simulink model "Assignment3_2_MMC"  (R2024b)
settings: Solver=VariableStepAuto  StartTime=0.0  StopTime=0.35  MaxStep=1e-5  RelTol=1e-3
values from neighbouring files (symbols this model uses):
  C_sm = 5e-3    (= 0.005)    [assignment3.m]    (also in matlab.mat)
libraries: spsIGBTDiodeLib x48, spsSeriesRLCBranchLib x30, spsVoltageMeasurementLib x25, spsTriangleGeneratorLib x24, spsCurrentMeasurementLib x9, slpidlib x5, spsabctodq0Lib x3, spsdq0toabcLib x2, spsDCVoltageSourceLib x1, eePowerMeasurement x1, spsThreePhaseSeriesRLCBranchLib x1, spsThreePhaseVIMeasurementLib x1
(part 1 of 2)
settings Model: Creator=alexapf.stu  LastModifiedBy=alexapf.stu
settings SolverCC: ZeroCrossAlgorithm=Adaptive
settings DebuggingCC: IgnoredZcDiagnostic=none

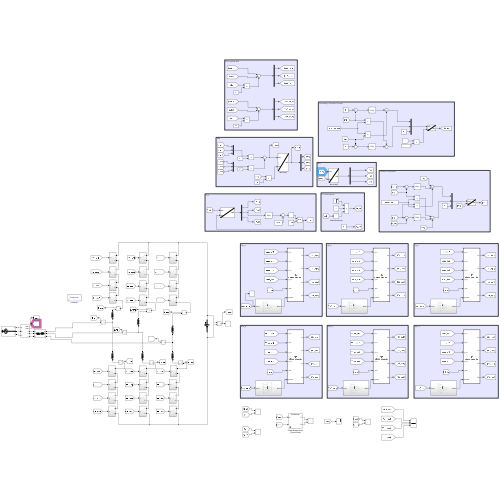
[thumbnail: Simulink's stored preview of the top-level diagram]
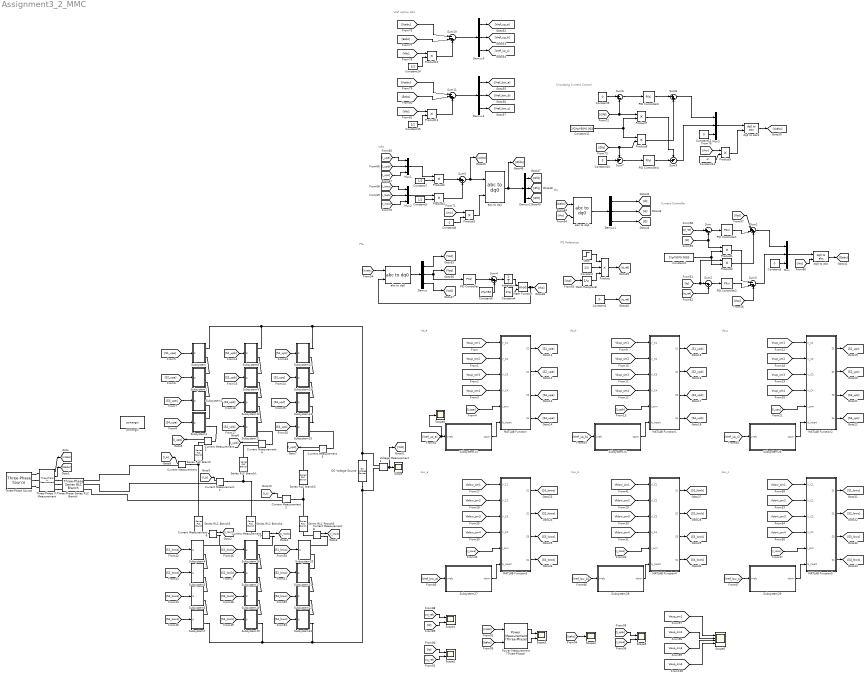
== system Assignment3_2_MMC ==
  note: Vref up/low abc
  note: Circulating Current Control
  note: izdq
  note: Idq
  note: Current Controller
  note: PQ Reference
  note: PLL
  note: Up_a
  note: Up_b
  note: Up_c
  note: low_c
  note: low_a
  note: low_b
  Constant : Constant  Value=2/3
  Constant{1,3,9..10,12} (5 alike) : Constant  Value=0
  Constant11 : Constant  Value=2*2*pi*50*0.003
  Constant13 : Constant  Value=-2
  Constant{5,7,14..15} (4 alike) : Constant  Value=1/2
  Constant2 : Constant  Value=2*pi*50*0.0083
  Constant4 : Constant  Value=2*pi
  Constant6 : Constant  Value=2*pi*50
  Constant8 : Constant  Value=-2
  Current Measurement{,1..8} (9 alike) : spsCurrentMeasurementLib/Current Measurement  PhasorSimulation=off  OutputType=Complex  PSBequivalent=0
  DC Voltage Source : spsDCVoltageSourceLib/DC Voltage Source  Amplitude=8e3  Measurements=None
  Demux{,1..4} (5 alike) : Demux  Outputs=3
  Integrator : Integrator
  MATLAB Function : MATLAB Function  TreatAsAtomicUnit=on
  MATLAB Function1 : MATLAB Function  TreatAsAtomicUnit=on
  MATLAB Function2 : MATLAB Function  TreatAsAtomicUnit=on
  MATLAB Function3 : MATLAB Function  TreatAsAtomicUnit=on
  MATLAB Function4 : MATLAB Function  TreatAsAtomicUnit=on
  MATLAB Function5 : MATLAB Function  TreatAsAtomicUnit=on
  Math Function : Math  Operator=mod
  Math Reciprocal : Math  Operator=reciprocal  SignedPower=on
  Mux{,1..3} (4 alike) : Mux  Inputs=3
  PID Controller : slpidlib/PID Controller  Controller=PI  Form=Parallel  TimeDomain=Continuous-time  UseExternalTs=off  SampleTime=-1  IntegratorMethod=Forward Euler  FilterMethod=Forward Euler  ControllerParametersSource=internal  P=0.0267  I=1.099  UseKiTs=off  D=0  UseExternalDerivativeSource=off  N=100  UseFilter=on  TunerSelectOption=Transfer Function Based (PID Tuner App)  InitialConditionSource=internal  InitialConditionForIntegrator=0  InitialConditionForFilter=0  DifferentiatorICPrevScaledInput=0  ExternalReset=none  TrackingMode=off  Kt=1  LimitOutput=off  SatLimitsSource=internal  UpperSaturationLimit=inf  LowerSaturationLimit=-inf  LinearizeAsGain=on  AntiWindupMode=none  Kb=1  LimitIntegrator=off  UpperIntegratorSaturationLimit=inf  LowerIntegratorSaturationLimit=-inf  POutMin=[]  POutMax=[]  IOutMin=[]  IOutMax=[]  DOutMin=[]  DOutMax=[]  NOutMin=[]  NOutMax=[]  SumOutMin=[]  SumOutMax=[]  SaturationOutMin=[]  SaturationOutMax=[]  PParamMin=[]  PParamMax=[]  IParamMin=[]  IParamMax=[]  DParamMin=[]  DParamMax=[]  NParamMin=[]  NParamMax=[]  KbParamMin=[]  KbParamMax=[]  KtParamMin=[]  KtParamMax=[]  KbOutMin=[]  KbOutMax=[]  KtOutMin=[]  KtOutMax=[]  IntegratorOutMin=[]  IntegratorOutMax=[]  FilterOutMin=[]  FilterOutMax=[]  SumI1OutMin=[]  SumI1OutMax=[]  SumI2OutMin=[]  SumI2OutMax=[]  SumI3OutMin=[]  SumI3OutMax=[]  SumI4OutMin=[]  SumI4OutMax=[]  SumDOutMin=[]  SumDOutMax=[]  DifferentiatorOutMin=[]  DifferentiatorOutMax=[]  FilterDiffOutCoefMin=[]  FilterDiffOutCoefMax=[]  ReciprocalOutMin=[]  ReciprocalOutMax=[]  SumDenOutMin=[]  SumDenOutMax=[]  SumNumOutMin=[]  SumNumOutMax=[]  DivideOutMin=[]  DivideOutMax=[]  UdiffTsProdOutMin=[]  UdiffTsProdOutMax=[]  NTsProdOutMin=[]  NTsProdOutMax=[]  UintegralTsProdOutMin=[]  UintegralTsProdOutMax=[]  UngainTsProdOutMin=[]  UngainTsProdOutMax=[]  ClampingZeroOutDataTypeStr=Inherit: Inherit via back propagation  ClampingZeroOutMin=[]  ClampingZeroOutMax=[]  FilterDenConstantOutDataTypeStr=Inherit: Inherit via back propagation  FilterDenConstantOutMin=[]  FilterDenConstantOutMax=[]  PCopyOutDataTypeStr=Inherit: Inherit via back propagation  PCopyOutMin=[]  PCopyOutMax=[]  NCopyOutDataTypeStr=Inherit: Inherit via back propagation  NCopyOutMin=[]  NCopyOutMax=[]  IntegratorContinuousStateAttributes=''  IntegratorStateMustResolveToSignalObject=off  IntegratorRTWStateStorageClass=Auto  FilterContinuousStateAttributes=''  FilterStateMustResolveToSignalObject=off  FilterRTWStateStorageClass=Auto  ParallelPVariant=InternalParameters  IdealPVariant=Disabled  IVariant=InternalParameters  DVariant=Disabled  IntegratorVariant=Continuous  SatVariant=Disabled  AWVariant=Passthrough  PCopyVariant=Disabled  TRVariant=Disabled  FdbkBlocksVariant=Forward  IdealPFdbkVariant=Disabled  SatFdbkVariant=Disabled  DerivativeFilterVariant=Disabled  NVariant=Disabled  NCopyVariant=Disabled_SignalSpec  FilterICVariant=Disabled  IntegratorICVariant=InternalICs  ExternalResetVariant=Disabled  TRSumVariant=Passthrough  SumFdbkVariant=Disabled  SumVariant=Sum_PI  TsampFilterVariant=InternalTs  TsampNgainVariant=Passthrough  TsampIntegralVariant=Disabled_SignalSpec  ExternalSaturationOutDataTypeStr=Inherit: Same as second input  DerivativeSourceVariant=Disabled  PreIntVariant=InternalPreInt
  PID Controller1 : slpidlib/PID Controller  Controller=PI  Form=Parallel  TimeDomain=Continuous-time  UseExternalTs=off  SampleTime=-1  IntegratorMethod=Forward Euler  FilterMethod=Forward Euler  ControllerParametersSource=internal  P=7.53  I=5.53  UseKiTs=off  D=0  UseExternalDerivativeSource=off  N=100  UseFilter=on  TunerSelectOption=Transfer Function Based (PID Tuner App)  InitialConditionSource=internal  InitialConditionForIntegrator=0  InitialConditionForFilter=0  DifferentiatorICPrevScaledInput=0  ExternalReset=none  TrackingMode=off  Kt=1  LimitOutput=off  SatLimitsSource=internal  UpperSaturationLimit=inf  LowerSaturationLimit=-inf  LinearizeAsGain=on  AntiWindupMode=none  Kb=1  LimitIntegrator=off  UpperIntegratorSaturationLimit=inf  LowerIntegratorSaturationLimit=-inf  POutMin=[]  POutMax=[]  IOutMin=[]  IOutMax=[]  DOutMin=[]  DOutMax=[]  NOutMin=[]  NOutMax=[]  SumOutMin=[]  SumOutMax=[]  SaturationOutMin=[]  SaturationOutMax=[]  PParamMin=[]  PParamMax=[]  IParamMin=[]  IParamMax=[]  DParamMin=[]  DParamMax=[]  NParamMin=[]  NParamMax=[]  KbParamMin=[]  KbParamMax=[]  KtParamMin=[]  KtParamMax=[]  KbOutMin=[]  KbOutMax=[]  KtOutMin=[]  KtOutMax=[]  IntegratorOutMin=[]  IntegratorOutMax=[]  FilterOutMin=[]  FilterOutMax=[]  SumI1OutMin=[]  SumI1OutMax=[]  SumI2OutMin=[]  SumI2OutMax=[]  SumI3OutMin=[]  SumI3OutMax=[]  SumI4OutMin=[]  SumI4OutMax=[]  SumDOutMin=[]  SumDOutMax=[]  DifferentiatorOutMin=[]  DifferentiatorOutMax=[]  FilterDiffOutCoefMin=[]  FilterDiffOutCoefMax=[]  ReciprocalOutMin=[]  ReciprocalOutMax=[]  SumDenOutMin=[]  SumDenOutMax=[]  SumNumOutMin=[]  SumNumOutMax=[]  DivideOutMin=[]  DivideOutMax=[]  UdiffTsProdOutMin=[]  UdiffTsProdOutMax=[]  NTsProdOutMin=[]  NTsProdOutMax=[]  UintegralTsProdOutMin=[]  UintegralTsProdOutMax=[]  UngainTsProdOutMin=[]  UngainTsProdOutMax=[]  ClampingZeroOutDataTypeStr=Inherit: Inherit via back propagation  ClampingZeroOutMin=[]  ClampingZeroOutMax=[]  FilterDenConstantOutDataTypeStr=Inherit: Inherit via back propagation  FilterDenConstantOutMin=[]  FilterDenConstantOutMax=[]  PCopyOutDataTypeStr=Inherit: Inherit via back propagation  PCopyOutMin=[]  PCopyOutMax=[]  NCopyOutDataTypeStr=Inherit: Inherit via back propagation  NCopyOutMin=[]  NCopyOutMax=[]  IntegratorContinuousStateAttributes=''  IntegratorStateMustResolveToSignalObject=off  IntegratorRTWStateStorageClass=Auto  FilterContinuousStateAttributes=''  FilterStateMustResolveToSignalObject=off  FilterRTWStateStorageClass=Auto  ParallelPVariant=InternalParameters  IdealPVariant=Disabled  IVariant=InternalParameters  DVariant=Disabled  IntegratorVariant=Continuous  SatVariant=Disabled  AWVariant=Passthrough  PCopyVariant=Disabled  TRVariant=Disabled  FdbkBlocksVariant=Forward  IdealPFdbkVariant=Disabled  SatFdbkVariant=Disabled  DerivativeFilterVariant=Disabled  NVariant=Disabled  NCopyVariant=Disabled_SignalSpec  FilterICVariant=Disabled  IntegratorICVariant=InternalICs  ExternalResetVariant=Disabled  TRSumVariant=Passthrough  SumFdbkVariant=Disabled  SumVariant=Sum_PI  TsampFilterVariant=InternalTs  TsampNgainVariant=Passthrough  TsampIntegralVariant=Disabled_SignalSpec  ExternalSaturationOutDataTypeStr=Inherit: Same as second input  DerivativeSourceVariant=Disabled  PreIntVariant=InternalPreInt
  PID Controller2 : slpidlib/PID Controller  Controller=PI  Form=Parallel  TimeDomain=Continuous-time  UseExternalTs=off  SampleTime=-1  IntegratorMethod=Forward Euler  FilterMethod=Forward Euler  ControllerParametersSource=internal  P=7.53  I=5.53  UseKiTs=off  D=0  UseExternalDerivativeSource=off  N=100  UseFilter=on  TunerSelectOption=Transfer Function Based (PID Tuner App)  InitialConditionSource=internal  InitialConditionForIntegrator=0  InitialConditionForFilter=0  DifferentiatorICPrevScaledInput=0  ExternalReset=none  TrackingMode=off  Kt=1  LimitOutput=off  SatLimitsSource=internal  UpperSaturationLimit=inf  LowerSaturationLimit=-inf  LinearizeAsGain=on  AntiWindupMode=none  Kb=1  LimitIntegrator=off  UpperIntegratorSaturationLimit=inf  LowerIntegratorSaturationLimit=-inf  POutMin=[]  POutMax=[]  IOutMin=[]  IOutMax=[]  DOutMin=[]  DOutMax=[]  NOutMin=[]  NOutMax=[]  SumOutMin=[]  SumOutMax=[]  SaturationOutMin=[]  SaturationOutMax=[]  PParamMin=[]  PParamMax=[]  IParamMin=[]  IParamMax=[]  DParamMin=[]  DParamMax=[]  NParamMin=[]  NParamMax=[]  KbParamMin=[]  KbParamMax=[]  KtParamMin=[]  KtParamMax=[]  KbOutMin=[]  KbOutMax=[]  KtOutMin=[]  KtOutMax=[]  IntegratorOutMin=[]  IntegratorOutMax=[]  FilterOutMin=[]  FilterOutMax=[]  SumI1OutMin=[]  SumI1OutMax=[]  SumI2OutMin=[]  SumI2OutMax=[]  SumI3OutMin=[]  SumI3OutMax=[]  SumI4OutMin=[]  SumI4OutMax=[]  SumDOutMin=[]  SumDOutMax=[]  DifferentiatorOutMin=[]  DifferentiatorOutMax=[]  FilterDiffOutCoefMin=[]  FilterDiffOutCoefMax=[]  ReciprocalOutMin=[]  ReciprocalOutMax=[]  SumDenOutMin=[]  SumDenOutMax=[]  SumNumOutMin=[]  SumNumOutMax=[]  DivideOutMin=[]  DivideOutMax=[]  UdiffTsProdOutMin=[]  UdiffTsProdOutMax=[]  NTsProdOutMin=[]  NTsProdOutMax=[]  UintegralTsProdOutMin=[]  UintegralTsProdOutMax=[]  UngainTsProdOutMin=[]  UngainTsProdOutMax=[]  ClampingZeroOutDataTypeStr=Inherit: Inherit via back propagation  ClampingZeroOutMin=[]  ClampingZeroOutMax=[]  FilterDenConstantOutDataTypeStr=Inherit: Inherit via back propagation  FilterDenConstantOutMin=[]  FilterDenConstantOutMax=[]  PCopyOutDataTypeStr=Inherit: Inherit via back propagation  PCopyOutMin=[]  PCopyOutMax=[]  NCopyOutDataTypeStr=Inherit: Inherit via back propagation  NCopyOutMin=[]  NCopyOutMax=[]  IntegratorContinuousStateAttributes=''  IntegratorStateMustResolveToSignalObject=off  IntegratorRTWStateStorageClass=Auto  FilterContinuousStateAttributes=''  FilterStateMustResolveToSignalObject=off  FilterRTWStateStorageClass=Auto  ParallelPVariant=InternalParameters  IdealPVariant=Disabled  IVariant=InternalParameters  DVariant=Disabled  IntegratorVariant=Continuous  SatVariant=Disabled  AWVariant=Passthrough  PCopyVariant=Disabled  TRVariant=Disabled  FdbkBlocksVariant=Forward  IdealPFdbkVariant=Disabled  SatFdbkVariant=Disabled  DerivativeFilterVariant=Disabled  NVariant=Disabled  NCopyVariant=Disabled_SignalSpec  FilterICVariant=Disabled  IntegratorICVariant=InternalICs  ExternalResetVariant=Disabled  TRSumVariant=Passthrough  SumFdbkVariant=Disabled  SumVariant=Sum_PI  TsampFilterVariant=InternalTs  TsampNgainVariant=Passthrough  TsampIntegralVariant=Disabled_SignalSpec  ExternalSaturationOutDataTypeStr=Inherit: Same as second input  DerivativeSourceVariant=Disabled  PreIntVariant=InternalPreInt
  PID Controller3 : slpidlib/PID Controller  Controller=PI  Form=Parallel  TimeDomain=Continuous-time  UseExternalTs=off  SampleTime=-1  IntegratorMethod=Forward Euler  FilterMethod=Forward Euler  ControllerParametersSource=internal  P=4  I=0  UseKiTs=off  D=0  UseExternalDerivativeSource=off  N=100  UseFilter=on  TunerSelectOption=Transfer Function Based (PID Tuner App)  InitialConditionSource=internal  InitialConditionForIntegrator=0  InitialConditionForFilter=0  DifferentiatorICPrevScaledInput=0  ExternalReset=none  TrackingMode=off  Kt=1  LimitOutput=off  SatLimitsSource=internal  UpperSaturationLimit=inf  LowerSaturationLimit=-inf  LinearizeAsGain=on  AntiWindupMode=none  Kb=1  LimitIntegrator=off  UpperIntegratorSaturationLimit=inf  LowerIntegratorSaturationLimit=-inf  POutMin=[]  POutMax=[]  IOutMin=[]  IOutMax=[]  DOutMin=[]  DOutMax=[]  NOutMin=[]  NOutMax=[]  SumOutMin=[]  SumOutMax=[]  SaturationOutMin=[]  SaturationOutMax=[]  PParamMin=[]  PParamMax=[]  IParamMin=[]  IParamMax=[]  DParamMin=[]  DParamMax=[]  NParamMin=[]  NParamMax=[]  KbParamMin=[]  KbParamMax=[]  KtParamMin=[]  KtParamMax=[]  KbOutMin=[]  KbOutMax=[]  KtOutMin=[]  KtOutMax=[]  IntegratorOutMin=[]  IntegratorOutMax=[]  FilterOutMin=[]  FilterOutMax=[]  SumI1OutMin=[]  SumI1OutMax=[]  SumI2OutMin=[]  SumI2OutMax=[]  SumI3OutMin=[]  SumI3OutMax=[]  SumI4OutMin=[]  SumI4OutMax=[]  SumDOutMin=[]  SumDOutMax=[]  DifferentiatorOutMin=[]  DifferentiatorOutMax=[]  FilterDiffOutCoefMin=[]  FilterDiffOutCoefMax=[]  ReciprocalOutMin=[]  ReciprocalOutMax=[]  SumDenOutMin=[]  SumDenOutMax=[]  SumNumOutMin=[]  SumNumOutMax=[]  DivideOutMin=[]  DivideOutMax=[]  UdiffTsProdOutMin=[]  UdiffTsProdOutMax=[]  NTsProdOutMin=[]  NTsProdOutMax=[]  UintegralTsProdOutMin=[]  UintegralTsProdOutMax=[]  UngainTsProdOutMin=[]  UngainTsProdOutMax=[]  ClampingZeroOutDataTypeStr=Inherit: Inherit via back propagation  ClampingZeroOutMin=[]  ClampingZeroOutMax=[]  FilterDenConstantOutDataTypeStr=Inherit: Inherit via back propagation  FilterDenConstantOutMin=[]  FilterDenConstantOutMax=[]  PCopyOutDataTypeStr=Inherit: Inherit via back propagation  PCopyOutMin=[]  PCopyOutMax=[]  NCopyOutDataTypeStr=Inherit: Inherit via back propagation  NCopyOutMin=[]  NCopyOutMax=[]  IntegratorContinuousStateAttributes=''  IntegratorStateMustResolveToSignalObject=off  IntegratorRTWStateStorageClass=Auto  FilterContinuousStateAttributes=''  FilterStateMustResolveToSignalObject=off  FilterRTWStateStorageClass=Auto  ParallelPVariant=InternalParameters  IdealPVariant=Disabled  IVariant=InternalParameters  DVariant=Disabled  IntegratorVariant=Continuous  SatVariant=Disabled  AWVariant=Passthrough  PCopyVariant=Disabled  TRVariant=Disabled  FdbkBlocksVariant=Forward  IdealPFdbkVariant=Disabled  SatFdbkVariant=Disabled  DerivativeFilterVariant=Disabled  NVariant=Disabled  NCopyVariant=Disabled_SignalSpec  FilterICVariant=Disabled  IntegratorICVariant=InternalICs  ExternalResetVariant=Disabled  TRSumVariant=Passthrough  SumFdbkVariant=Disabled  SumVariant=Sum_PI  TsampFilterVariant=InternalTs  TsampNgainVariant=Passthrough  TsampIntegralVariant=Disabled_SignalSpec  ExternalSaturationOutDataTypeStr=Inherit: Same as second input  DerivativeSourceVariant=Disabled  PreIntVariant=InternalPreInt
  PID Controller4 : slpidlib/PID Controller  Controller=PI  Form=Parallel  TimeDomain=Continuous-time  UseExternalTs=off  SampleTime=-1  IntegratorMethod=Forward Euler  FilterMethod=Forward Euler  ControllerParametersSource=internal  P=4  I=0  UseKiTs=off  D=0  UseExternalDerivativeSource=off  N=100  UseFilter=on  TunerSelectOption=Transfer Function Based (PID Tuner App)  InitialConditionSource=internal  InitialConditionForIntegrator=0  InitialConditionForFilter=0  DifferentiatorICPrevScaledInput=0  ExternalReset=none  TrackingMode=off  Kt=1  LimitOutput=off  SatLimitsSource=internal  UpperSaturationLimit=inf  LowerSaturationLimit=-inf  LinearizeAsGain=on  AntiWindupMode=none  Kb=1  LimitIntegrator=off  UpperIntegratorSaturationLimit=inf  LowerIntegratorSaturationLimit=-inf  POutMin=[]  POutMax=[]  IOutMin=[]  IOutMax=[]  DOutMin=[]  DOutMax=[]  NOutMin=[]  NOutMax=[]  SumOutMin=[]  SumOutMax=[]  SaturationOutMin=[]  SaturationOutMax=[]  PParamMin=[]  PParamMax=[]  IParamMin=[]  IParamMax=[]  DParamMin=[]  DParamMax=[]  NParamMin=[]  NParamMax=[]  KbParamMin=[]  KbParamMax=[]  KtParamMin=[]  KtParamMax=[]  KbOutMin=[]  KbOutMax=[]  KtOutMin=[]  KtOutMax=[]  IntegratorOutMin=[]  IntegratorOutMax=[]  FilterOutMin=[]  FilterOutMax=[]  SumI1OutMin=[]  SumI1OutMax=[]  SumI2OutMin=[]  SumI2OutMax=[]  SumI3OutMin=[]  SumI3OutMax=[]  SumI4OutMin=[]  SumI4OutMax=[]  SumDOutMin=[]  SumDOutMax=[]  DifferentiatorOutMin=[]  DifferentiatorOutMax=[]  FilterDiffOutCoefMin=[]  FilterDiffOutCoefMax=[]  ReciprocalOutMin=[]  ReciprocalOutMax=[]  SumDenOutMin=[]  SumDenOutMax=[]  SumNumOutMin=[]  SumNumOutMax=[]  DivideOutMin=[]  DivideOutMax=[]  UdiffTsProdOutMin=[]  UdiffTsProdOutMax=[]  NTsProdOutMin=[]  NTsProdOutMax=[]  UintegralTsProdOutMin=[]  UintegralTsProdOutMax=[]  UngainTsProdOutMin=[]  UngainTsProdOutMax=[]  ClampingZeroOutDataTypeStr=Inherit: Inherit via back propagation  ClampingZeroOutMin=[]  ClampingZeroOutMax=[]  FilterDenConstantOutDataTypeStr=Inherit: Inherit via back propagation  FilterDenConstantOutMin=[]  FilterDenConstantOutMax=[]  PCopyOutDataTypeStr=Inherit: Inherit via back propagation  PCopyOutMin=[]  PCopyOutMax=[]  NCopyOutDataTypeStr=Inherit: Inherit via back propagation  NCopyOutMin=[]  NCopyOutMax=[]  IntegratorContinuousStateAttributes=''  IntegratorStateMustResolveToSignalObject=off  IntegratorRTWStateStorageClass=Auto  FilterContinuousStateAttributes=''  FilterStateMustResolveToSignalObject=off  FilterRTWStateStorageClass=Auto  ParallelPVariant=InternalParameters  IdealPVariant=Disabled  IVariant=InternalParameters  DVariant=Disabled  IntegratorVariant=Continuous  SatVariant=Disabled  AWVariant=Passthrough  PCopyVariant=Disabled  TRVariant=Disabled  FdbkBlocksVariant=Forward  IdealPFdbkVariant=Disabled  SatFdbkVariant=Disabled  DerivativeFilterVariant=Disabled  NVariant=Disabled  NCopyVariant=Disabled_SignalSpec  FilterICVariant=Disabled  IntegratorICVariant=InternalICs  ExternalResetVariant=Disabled  TRSumVariant=Passthrough  SumFdbkVariant=Disabled  SumVariant=Sum_PI  TsampFilterVariant=InternalTs  TsampNgainVariant=Passthrough  TsampIntegralVariant=Disabled_SignalSpec  ExternalSaturationOutDataTypeStr=Inherit: Same as second input  DerivativeSourceVariant=Disabled  PreIntVariant=InternalPreInt
  Power Measurement (Three-Phase) : eePowerMeasurement/Power Measurement (Three-Phase)  LabelModeActiveChoice=Continuous  F=60  K=[1]  Seq=Positive  Ts=0
  Product : Product  Inputs=3
  Product{1..5,7..11} (10 alike) : Product
  Scope : Scope
  Scope{1..3,5} (4 alike) : Scope  NumInputPorts=2
  Scope4 : Scope
  Scope6 : Scope  NumInputPorts=4
  Scope8 : Scope
  Series RLC Branch{,1..5} (6 alike) : spsSeriesRLCBranchLib/Series RLC Branch  LConnTagsString=__new0  RConnTagsString=__new0  BranchType=L  Resistance=0  Inductance=3e-3  SetiL0=off  InitialCurrent=0  Capacitance=0  Setx0=off  InitialVoltage=0  Measurements=None
  Step : Step  Time=0.05  After=1e6  SampleTime=0.0001
  Subsystem : Subsystem
  Subsystem1 : Subsystem
  Subsystem10 : Subsystem
  Subsystem11 : Subsystem
  Subsystem12 : Subsystem
  Subsystem13 : Subsystem
  Subsystem14 : Subsystem
  Subsystem15 : Subsystem
  Subsystem16 : Subsystem
  Subsystem17 : Subsystem
  Subsystem18 : Subsystem
  Subsystem19 : Subsystem
  Subsystem2 : Subsystem
  Subsystem20 : Subsystem
  Subsystem21 : Subsystem
  Subsystem22 : Subsystem
  Subsystem23 : Subsystem
  Subsystem24 : Subsystem
  Subsystem25 : Subsystem
  Subsystem26 : Subsystem
  Subsystem27 : Subsystem
  Subsystem28 : Subsystem
  Subsystem29 : Subsystem
  Subsystem3 : Subsystem
  Subsystem4 : Subsystem
  Subsystem5 : Subsystem
  Subsystem6 : Subsystem
  Subsystem7 : Subsystem
  Subsystem8 : Subsystem
  Subsystem9 : Subsystem
  Sum : Sum  Inputs=|+-
  Sum1 : Sum  Inputs=|+-+
  Sum10 : Sum  Inputs=|--+
  Sum11 : Sum  Inputs=|-++
  Sum2 : Sum  Inputs=|-+
  Sum3 : Sum  Inputs=|--+
  Sum4 : Sum  Inputs=|++
  Sum5 : Sum  Inputs=|++
  Sum6 : Sum  Inputs=|+-
  Sum7 : Sum  Inputs=-+|
  Sum8 : Sum  Inputs=|++
  Sum9 : Sum  Inputs=-+|
  Three-Phase Series RLC Branch : spsThreePhaseSeriesRLCBranchLib/Three-Phase Series RLC Branch  LConnTagsString=A|B|C  RConnTagsString=A|B|C  BranchType=RL  Resistance=8.3e-3  Inductance=8.3e-3  Capacitance=1e-6  Measurements=Branch voltages and currents
  Three-Phase V-I Measurement : spsThreePhaseVIMeasurementLib/Three-Phase V-I Measurement  VoltageMeasurement=phase-to-ground  SetLabelV=off  LabelV=Vabc  Vpu=off  VpuLL=off  CurrentMeasurement=yes  SetLabelI=off  LabelI=Iabc  Ipu=off  Pbase=100e6  Vbase=500e3  OutputType=Complex  PhasorSimulation=off  PSBequivalent=0
  Three-Phase Source : spsThreePhaseSourceLib/Three-Phase Source  InternalConnection=Yg  VoltagePhases=off  Voltage=4160  PhaseAngle=0  Voltage_phases=[25e3 25e3 25e3]/sqrt(3)  PhaseAngles_phases=[0 -120 +120]  Frequency=50  NonIdealSource=off  SpecifyImpedance=off  Resistance=0.8929  Inductance=16.58e-3  ShortCircuitLevel=100e6  BaseVoltage=25e3  XRratio=7  BusType=swing  Pref=10e3  Qref=0  Prefabc=[10e3, 10e3, 10e3]  Qrefabc=[0, 0, 0]  Qmin=-inf  Qmax=inf
  Voltage Measurement3 : spsVoltageMeasurementLib/Voltage Measurement  PhasorSimulation=off  OutputType=Complex  PSBequivalent=0
  abc to dq0 : spsabctodq0Lib/abc to dq0  Alignment=90 degrees behind phase A axis
  abc to dq1 : spsabctodq0Lib/abc to dq0  Alignment=90 degrees behind phase A axis
  abc to dq2 : spsabctodq0Lib/abc to dq0  Alignment=90 degrees behind phase A axis
  dq0 to abc : spsdq0toabcLib/dq0 to abc  Alignment=90 degrees behind phase A axis
  dq0 to abc1 : spsdq0toabcLib/dq0 to abc  Alignment=90 degrees behind phase A axis
  powergui : spspowerguiLib/powergui  Priority=1  SimulationMode=Continuous  SampleTime=50e-6  frequency=60  Iterations=50  frequencyindice=50  Pbase=100e6  ErrMax=1e-4  UnitsV=kV  UnitsW=MW  buscounter=0  FunctionMessages=off  echomessages=off  EnableUseOfTLC=off  CurrentSourceSwitches=off  DisableSnubberDevices=off  DisableRonSwitches=off  DisableVfSwitches=off  DisplayEquations=off  AutomaticDiscreteSolvers=off  SolverType=Tustin/Backward Euler (TBE)  Interpol=off  ExternalGateDelay=off  methode=off  Ts=100  x0status=blocks  SPID=on  SwTol=0  HookPort=off  NonlinearTolerance=1e-4  nMaxIteration=100  ContinueOnMaxIteration=off  RestoreLinks=warning  ResistiveCurrentMeasurement=off  Frange=[0:2:500]  Ylog=off  Xlog=on  ShowGrid=off  save=off  variable=ZData  structure=0  ZoomFFT=off  StartTime=0.0  cycles=1  DisplayStyle=1  fundamental=60  FreqAxis=off  MaxFrequency=1000  frequencyindicesteady=1  RmsSteady=1  display=off
  wires:
  Three-Phase V-I Measurement/1 -> [Vsabc]
  Three-Phase V-I Measurement/2 -> [Isabc]
  Current Measurement6/1 -> [I_lowa]
  Current Measurement7/1 -> [I_lowb]
  Current Measurement8/1 -> [I_lowc]
  Current Measurement3/1 -> [I_upa]
  Current Measurement4/1 -> [I_upb]
  Current Measurement5/1 -> [I_upc]
  Current Measurement/1 -> [I_a]
  Current Measurement1/1 -> [I_b]
  Current Measurement2/1 -> [I_c]
  [S1_upa] -> Subsystem/1(g)
  [S2_upa] -> Subsystem1/1(g)
  [S3_upa] -> Subsystem2/1(g)
  [S4_upa] -> Subsystem3/1(g)
  [I_upa] -> MATLAB Function/5(i_arm)
  MATLAB Function/1(S1) -> [S1_upa]
  MATLAB Function/4(S4) -> [S4_upa]
  [Vaup_sm2] -> MATLAB Function/2(V_C2)
  [Vaup_sm4] -> MATLAB Function/4(V_C4)
  Subsystem24/1(Narm) -> MATLAB Function/6(N_insert)
  [Vaup_sm3] -> MATLAB Function/3(V_C3)
  [Vaup_sm1] -> MATLAB Function/1(V_C1)
  MATLAB Function/2(S2) -> [S2_upa]
  MATLAB Function/3(S3) -> [S3_upa]
  [Vref_up_a] -> Scope8/1, Subsystem24/1(Vref,j)
  [I_upb] -> MATLAB Function1/5(i_arm)
  [Vbup_sm2] -> MATLAB Function1/2(V_C2)
  [Vbup_sm4] -> MATLAB Function1/4(V_C4)
  Subsystem25/1(Narm) -> MATLAB Function1/6(N_insert)
  MATLAB Function1/1(S1) -> [S1_upb]
  [Vbup_sm3] -> MATLAB Function1/3(V_C3)
  MATLAB Function1/2(S2) -> [S2_upb]
  [Vbup_sm1] -> MATLAB Function1/1(V_C1)
  [Vref_up_b] -> Subsystem25/1(Vref,j)
  MATLAB Function1/4(S4) -> [S4_upb]
  MATLAB Function1/3(S3) -> [S3_upb]
  [S1_upb] -> Subsystem8/1(g)
  [S2_upb] -> Subsystem9/1(g)
  [S3_upb] -> Subsystem10/1(g)
  [S4_upb] -> Subsystem11/1(g)
  MATLAB Function2/4(S4) -> [S4_upc]
  [Vcup_sm2] -> MATLAB Function2/2(V_C2)
  MATLAB Function2/3(S3) -> [S3_upc]
  MATLAB Function2/1(S1) -> [S1_upc]
  [Vcup_sm1] -> MATLAB Function2/1(V_C1)
  Subsystem26/1(Narm) -> MATLAB Function2/6(N_insert)
  MATLAB Function2/2(S2) -> [S2_upc]
  [I_upc] -> MATLAB Function2/5(i_arm)
  [Vcup_sm3] -> MATLAB Function2/3(V_C3)
  [Vref_up_c] -> Subsystem26/1(Vref,j)
  [Vcup_sm4] -> MATLAB Function2/4(V_C4)
  [S1_upc] -> Subsystem12/1(g)
  [S2_upc] -> Subsystem13/1(g)
  [S3_upc] -> Subsystem14/1(g)
  [S4_upc] -> Subsystem15/1(g)
  [I_lowa] -> MATLAB Function3/5(i_arm)
  [Valow_sm2] -> MATLAB Function3/2(V_C2)
  Subsystem27/1(Narm) -> MATLAB Function3/6(N_insert)
  MATLAB Function3/1(S1) -> [S1_lowa]
  [Valow_sm3] -> MATLAB Function3/3(V_C3)
  MATLAB Function4/1(S1) -> [S1_lowb]
  Subsystem28/1(Narm) -> MATLAB Function4/6(N_insert)
  [Vclow_sm3] -> MATLAB Function5/3(V_C3)
  MATLAB Function4/3(S3) -> [S3_lowb]
  MATLAB Function5/2(S2) -> [S2_lowc]
  [Valow_sm4] -> MATLAB Function3/4(V_C4)
  [Vblow_sm4] -> MATLAB Function4/4(V_C4)
  [Vref_low_c] -> Subsystem29/1(Vref,j)
  MATLAB Function4/4(S4) -> [S4_lowb]
  [I_lowc] -> MATLAB Function5/5(i_arm)
  [Vblow_sm3] -> MATLAB Function4/3(V_C3)
  [Valow_sm1] -> MATLAB Function3/1(V_C1)
  MATLAB Function3/3(S3) -> [S3_lowa]
  [I_lowb] -> MATLAB Function4/5(i_arm)
  [Vblow_sm2] -> MATLAB Function4/2(V_C2)
  MATLAB Function3/2(S2) -> [S2_lowa]
  [Vref_low_b] -> Subsystem28/1(Vref,j)
  [Vblow_sm1] -> MATLAB Function4/1(V_C1)
  MATLAB Function4/2(S2) -> [S2_lowb]
  [Vclow_sm1] -> MATLAB Function5/1(V_C1)
  Subsystem29/1(Narm) -> MATLAB Function5/6(N_insert)
  MATLAB Function5/3(S3) -> [S3_lowc]
  [Vclow_sm2] -> MATLAB Function5/2(V_C2)
  MATLAB Function5/4(S4) -> [S4_lowc]
  MATLAB Function5/1(S1) -> [S1_lowc]
  [Vclow_sm4] -> MATLAB Function5/4(V_C4)
  [Vref_low_a] -> Subsystem27/1(Vref,j)
  MATLAB Function3/4(S4) -> [S4_lowa]
  [S2_lowa] -> Subsystem5/1(g)
  [S1_lowa] -> Subsystem4/1(g)
  [S4_lowa] -> Subsystem7/1(g)
  [S3_lowa] -> Subsystem6/1(g)
  [S2_lowb] -> Subsystem17/1(g)
  [S4_lowb] -> Subsystem19/1(g)
  [S1_lowb] -> Subsystem16/1(g)
  [S3_lowb] -> Subsystem18/1(g)
  [S1_lowc] -> Subsystem20/1(g)
  [S2_lowc] -> Subsystem21/1(g)
  [S3_lowc] -> Subsystem22/1(g)
  [S4_lowc] -> Subsystem23/1(g)
  Constant4/1 -> Math Function/2
  Constant6/1 -> Sum4/2
  [Vsabc] -> abc to dq0/1
  Demux/1 -> [Vsd]
  abc to dq0/1 -> Demux/1
  Demux/3 -> [Vs0]
  Sum4/1 -> Integrator/1
  PID Controller/1 -> Sum4/1
  Demux/2 -> [Vsq], PID Controller/1
  Integrator/1 -> Math Function/1
  Math Function/1 -> abc to dq0/2, [rho]
  Math Reciprocal/1 -> Product/3
  Step/1 -> Product/1
  Constant/1 -> Product/2
  Product/1 -> [Id_ref]
  [Vsd] -> Math Reciprocal/1
  Constant1/1 -> [Iq_ref]
  [rho] -> dq0 to abc/2
  [Vsd] -> Sum1/1
  [Iq_ref] -> Sum2/2
  [Id_ref] -> Sum/1
  Sum1/1 -> Mux/1
  Product2/1 -> Sum1/3
  Sum2/1 -> PID Controller2/1
  Constant3/1 -> Mux/3
  [Id] -> Product1/1, Sum/2
  Product1/1 -> Sum3/1
  Sum/1 -> PID Controller1/1
  Sum3/1 -> Mux/2
  PID Controller2/1 -> Sum3/2
  Mux/1 -> dq0 to abc/1
  dq0 to abc/1 -> [Eabc]
  [Vsq] -> Sum3/3
  PID Controller1/1 -> Sum1/2
  Constant2/1 -> Product1/2, Product2/2
  [Iq] -> Product2/1, Sum2/1
  [rho] -> abc to dq2/2
  Demux1/1 -> [Id]
  abc to dq2/1 -> Demux1/1
  Demux1/3 -> [I0]
  [Isabc] -> abc to dq2/1
  Demux1/2 -> [Iq]
  [I_upa] -> Mux1/1
  [I_lowc] -> Mux2/3
  [I_lowa] -> Mux2/1
  [I_upb] -> Mux1/2
  [I_lowb] -> Mux2/2
  Mux2/1 -> Product4/1
  Mux1/1 -> Product3/1
  Constant8/1 -> Product5/2
  Constant7/1 -> Product3/2
  Sum5/1 -> [izabc], abc to dq1/1
  Product3/1 -> Sum5/1
  [I_upc] -> Mux1/3
  [rho] -> Product5/1
  Product5/1 -> abc to dq1/2
  abc to dq1/1 -> Demux2/1, [i2fdq]
  Constant5/1 -> Product4/2
  Product4/1 -> Sum5/2
  Demux2/1 -> [i2fd]
  Demux2/2 -> [i2fq]
  Demux2/3 -> [i2f0]
  Product8/1 -> Sum8/2
  Sum7/1 -> PID Controller4/1
  Sum9/1 -> Mux3/2
  Constant13/1 -> Product9/2
  dq0 to abc1/1 -> [Vzabc]
  Constant12/1 -> Mux3/3
  PID Controller3/1 -> Sum8/1
  Mux3/1 -> dq0 to abc1/1
  Product9/1 -> dq0 to abc1/2
  Constant9/1 -> Sum6/1
  [rho] -> Product9/1
  Sum6/1 -> PID Controller3/1
  [i2fd] -> Product7/1, Sum6/2
  Sum8/1 -> Mux3/1
  [i2fq] -> Sum7/1, Product8/2
  Voltage Measurement3/1 -> [Vdc], Scope/1
  Demux3/1 -> [Vref_up_a]
  Demux3/2 -> [Vref_up_b]
  [Eabc] -> Sum10/2
  [Vdc] -> Product11/1
  [Vzabc] -> Sum11/1
  Product11/1 -> Sum11/3
  [Eabc] -> Sum11/2
  Constant15/1 -> Product11/2
  Demux4/3 -> [Vref_low_c]
  Demux4/1 -> [Vref_low_a]
  Demux4/2 -> [Vref_low_b]
  [Vzabc] -> Sum10/1
  Sum11/1 -> Demux4/1
  Demux3/3 -> [Vref_up_c]
  Product10/1 -> Sum10/3
  Constant14/1 -> Product10/2
  [Vdc] -> Product10/1
  Sum10/1 -> Demux3/1
  [Id_ref] -> Scope1/1
  [Id] -> Scope1/2
  [Iq] -> Scope2/1
  [Iq_ref] -> Scope2/2
  [Vsabc] -> Power Measurement (Three-Phase)/1
  Power Measurement (Three-Phase)/1 -> Scope3/1
  Power Measurement (Three-Phase)/2 -> Scope3/2
  [Isabc] -> Power Measurement (Three-Phase)/2
  [izabc] -> Scope4/1
  [I_upa] -> Scope5/1
  [I_lowa] -> Scope5/2
  [Vaup_sm1] -> Scope6/1
  [Vaup_sm3] -> Scope6/3
  [Vaup_sm2] -> Scope6/2
  [Vaup_sm4] -> Scope6/4
  Constant11/1 -> Product8/1, Product7/2
  PID Controller4/1 -> Sum9/2
  Product7/1 -> Sum9/1
  Constant10/1 -> Sum7/2
  connections:
  Subsystem1/RConn1 -- Subsystem/RConn2
  Subsystem2/RConn1 -- Subsystem1/RConn2
  Subsystem3/RConn1 -- Subsystem2/RConn2
  Series RLC Branch5/LConn1 -- Current Measurement2/LConn1 -- Series RLC Branch2/RConn1
  Current Measurement/RConn1 -- Three-Phase Series RLC Branch/RConn1
  Subsystem9/RConn1 -- Subsystem8/RConn2
  Subsystem10/RConn1 -- Subsystem9/RConn2
  Subsystem11/RConn1 -- Subsystem10/RConn2
  Subsystem13/RConn1 -- Subsystem12/RConn2
  Subsystem14/RConn1 -- Subsystem13/RConn2
  Subsystem15/RConn1 -- Subsystem14/RConn2
  Subsystem5/RConn1 -- Subsystem4/RConn2
  Subsystem6/RConn1 -- Subsystem5/RConn2
  Subsystem7/RConn1 -- Subsystem6/RConn2
  Subsystem19/RConn1 -- Subsystem18/RConn2
  Subsystem17/RConn1 -- Subsystem16/RConn2
  Subsystem18/RConn1 -- Subsystem17/RConn2
  Subsystem23/RConn1 -- Subsystem22/RConn2
  Subsystem21/RConn1 -- Subsystem20/RConn2
  Subsystem22/RConn1 -- Subsystem21/RConn2
  DC Voltage Source/RConn1 -- Subsystem12/RConn1 -- Subsystem8/RConn1 -- Subsystem/RConn1 -- Voltage Measurement3/LConn1
  DC Voltage Source/LConn1 -- Voltage Measurement3/LConn2 -- Subsystem23/RConn2 -- Subsystem19/RConn2 -- Subsystem7/RConn2
  Three-Phase V-I Measurement/RConn3 -- Three-Phase Series RLC Branch/LConn3
  Three-Phase Source/RConn2 -- Three-Phase V-I Measurement/LConn2
  Three-Phase V-I Measurement/RConn2 -- Three-Phase Series RLC Branch/LConn2
  Three-Phase Source/RConn1 -- Three-Phase V-I Measurement/LConn1
  Three-Phase V-I Measurement/RConn1 -- Three-Phase Series RLC Branch/LConn1
  Three-Phase Source/RConn3 -- Three-Phase V-I Measurement/LConn3
  Series RLC Branch1/RConn1 -- Current Measurement1/LConn1 -- Series RLC Branch4/LConn1
  Series RLC Branch3/LConn1 -- Current Measurement/LConn1 -- Series RLC Branch/RConn1
  Current Measurement1/RConn1 -- Three-Phase Series RLC Branch/RConn2
  Current Measurement2/RConn1 -- Three-Phase Series RLC Branch/RConn3
  Subsystem3/RConn2 -- Current Measurement3/LConn1
  Current Measurement3/RConn1 -- Series RLC Branch/LConn1
  Current Measurement4/LConn1 -- Subsystem11/RConn2
  Current Measurement4/RConn1 -- Series RLC Branch1/LConn1
  Current Measurement5/LConn1 -- Subsystem15/RConn2
  Current Measurement5/RConn1 -- Series RLC Branch2/LConn1
  Current Measurement6/LConn1 -- Series RLC Branch3/RConn1
  Current Measurement6/RConn1 -- Subsystem4/RConn1
  Current Measurement7/LConn1 -- Series RLC Branch4/RConn1
  Current Measurement7/RConn1 -- Subsystem16/RConn1
  Series RLC Branch5/RConn1 -- Current Measurement8/LConn1
  Current Measurement8/RConn1 -- Subsystem20/RConn1

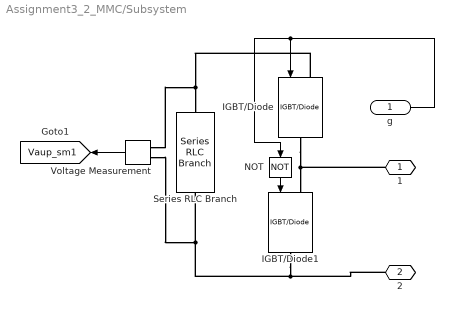
== system Assignment3_2_MMC/Subsystem ==
  g : Inport
  IGBT/Diode : spsIGBTDiodeLib/IGBT//Diode  Ron=1e-3  Rs=1e5  Cs=inf  Measurements=off
  IGBT/Diode1 : spsIGBTDiodeLib/IGBT//Diode  Ron=1e-3  Rs=1e5  Cs=inf  Measurements=off
  NOT : Logic  Operator=NOT  IconShape=distinctive  AllPortsSameDT=off  OutDataTypeStr=boolean
  Series RLC Branch : spsSeriesRLCBranchLib/Series RLC Branch  LConnTagsString=__new0  RConnTagsString=__new0  BranchType=C  Resistance=1  Inductance=1e-3  SetiL0=off  InitialCurrent=0  Capacitance=C_sm  Setx0=on  InitialVoltage=V_sm  Measurements=None
  Voltage Measurement : spsVoltageMeasurementLib/Voltage Measurement  PhasorSimulation=off  OutputType=Complex  PSBequivalent=0
  1 : PMIOPort  Side=Right
  2 : PMIOPort  Port=2  Side=Right
  tag scope: Vaup_sm1=global
  wires:
  NOT/1 -> IGBT/Diode1/1
  g/1 -> IGBT/Diode/1, NOT/1
  Voltage Measurement/1 -> [Vaup_sm1]
  connections:
  IGBT/Diode/RConn1 -- IGBT/Diode1/LConn1 -- 1/RConn1
  IGBT/Diode/LConn1 -- Voltage Measurement/LConn1 -- Series RLC Branch/LConn1
  IGBT/Diode1/RConn1 -- 2/RConn1 -- Voltage Measurement/LConn2 -- Series RLC Branch/RConn1

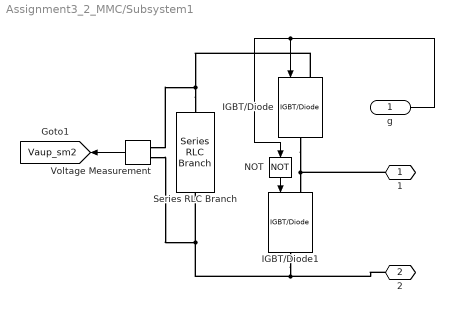
== system Assignment3_2_MMC/Subsystem1 ==
  g : Inport
  IGBT/Diode : spsIGBTDiodeLib/IGBT//Diode  Ron=1e-3  Rs=1e5  Cs=inf  Measurements=off
  IGBT/Diode1 : spsIGBTDiodeLib/IGBT//Diode  Ron=1e-3  Rs=1e5  Cs=inf  Measurements=off
  NOT : Logic  Operator=NOT  IconShape=distinctive  AllPortsSameDT=off  OutDataTypeStr=boolean
  Series RLC Branch : spsSeriesRLCBranchLib/Series RLC Branch  LConnTagsString=__new0  RConnTagsString=__new0  BranchType=C  Resistance=1  Inductance=1e-3  SetiL0=off  InitialCurrent=0  Capacitance=C_sm  Setx0=on  InitialVoltage=V_sm  Measurements=None
  Voltage Measurement : spsVoltageMeasurementLib/Voltage Measurement  PhasorSimulation=off  OutputType=Complex  PSBequivalent=0
  1 : PMIOPort  Side=Right
  2 : PMIOPort  Port=2  Side=Right
  tag scope: Vaup_sm2=global
  wires:
  NOT/1 -> IGBT/Diode1/1
  g/1 -> IGBT/Diode/1, NOT/1
  Voltage Measurement/1 -> [Vaup_sm2]
  connections:
  IGBT/Diode/RConn1 -- 1/RConn1 -- IGBT/Diode1/LConn1
  Series RLC Branch/LConn1 -- IGBT/Diode/LConn1 -- Voltage Measurement/LConn1
  Series RLC Branch/RConn1 -- 2/RConn1 -- IGBT/Diode1/RConn1 -- Voltage Measurement/LConn2

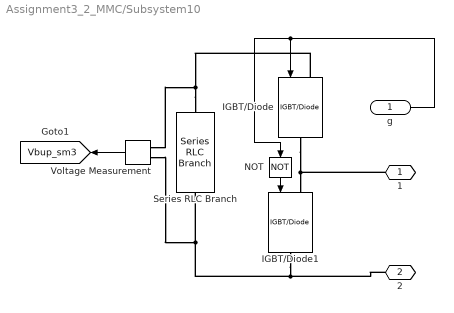
== system Assignment3_2_MMC/Subsystem10 ==
  g : Inport
  IGBT/Diode : spsIGBTDiodeLib/IGBT//Diode  Ron=1e-3  Rs=1e5  Cs=inf  Measurements=off
  IGBT/Diode1 : spsIGBTDiodeLib/IGBT//Diode  Ron=1e-3  Rs=1e5  Cs=inf  Measurements=off
  NOT : Logic  Operator=NOT  IconShape=distinctive  AllPortsSameDT=off  OutDataTypeStr=boolean
  Series RLC Branch : spsSeriesRLCBranchLib/Series RLC Branch  LConnTagsString=__new0  RConnTagsString=__new0  BranchType=C  Resistance=1  Inductance=1e-3  SetiL0=off  InitialCurrent=0  Capacitance=C_sm  Setx0=on  InitialVoltage=V_sm  Measurements=None
  Voltage Measurement : spsVoltageMeasurementLib/Voltage Measurement  PhasorSimulation=off  OutputType=Complex  PSBequivalent=0
  1 : PMIOPort  Side=Right
  2 : PMIOPort  Port=2  Side=Right
  tag scope: Vbup_sm3=global
  wires:
  NOT/1 -> IGBT/Diode1/1
  g/1 -> IGBT/Diode/1, NOT/1
  Voltage Measurement/1 -> [Vbup_sm3]
  connections:
  IGBT/Diode/RConn1 -- 1/RConn1 -- IGBT/Diode1/LConn1
  Series RLC Branch/LConn1 -- IGBT/Diode/LConn1 -- Voltage Measurement/LConn1
  Series RLC Branch/RConn1 -- 2/RConn1 -- IGBT/Diode1/RConn1 -- Voltage Measurement/LConn2

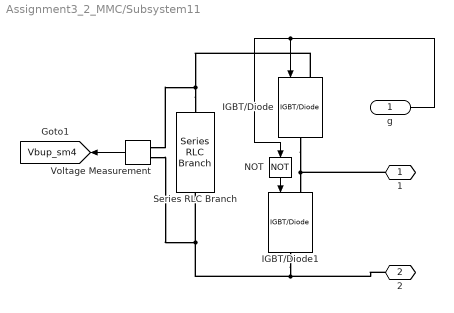
== system Assignment3_2_MMC/Subsystem11 ==
  g : Inport
  IGBT/Diode : spsIGBTDiodeLib/IGBT//Diode  Ron=1e-3  Rs=1e5  Cs=inf  Measurements=off
  IGBT/Diode1 : spsIGBTDiodeLib/IGBT//Diode  Ron=1e-3  Rs=1e5  Cs=inf  Measurements=off
  NOT : Logic  Operator=NOT  IconShape=distinctive  AllPortsSameDT=off  OutDataTypeStr=boolean
  Series RLC Branch : spsSeriesRLCBranchLib/Series RLC Branch  LConnTagsString=__new0  RConnTagsString=__new0  BranchType=C  Resistance=1  Inductance=1e-3  SetiL0=off  InitialCurrent=0  Capacitance=C_sm  Setx0=on  InitialVoltage=V_sm  Measurements=None
  Voltage Measurement : spsVoltageMeasurementLib/Voltage Measurement  PhasorSimulation=off  OutputType=Complex  PSBequivalent=0
  1 : PMIOPort  Side=Right
  2 : PMIOPort  Port=2  Side=Right
  tag scope: Vbup_sm4=global
  wires:
  NOT/1 -> IGBT/Diode1/1
  g/1 -> IGBT/Diode/1, NOT/1
  Voltage Measurement/1 -> [Vbup_sm4]
  connections:
  IGBT/Diode/RConn1 -- 1/RConn1 -- IGBT/Diode1/LConn1
  Series RLC Branch/LConn1 -- IGBT/Diode/LConn1 -- Voltage Measurement/LConn1
  Series RLC Branch/RConn1 -- 2/RConn1 -- IGBT/Diode1/RConn1 -- Voltage Measurement/LConn2

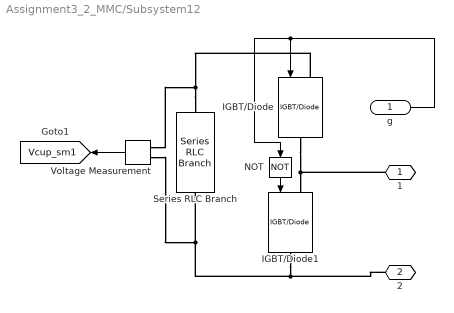
== system Assignment3_2_MMC/Subsystem12 ==
  g : Inport
  IGBT/Diode : spsIGBTDiodeLib/IGBT//Diode  Ron=1e-3  Rs=1e5  Cs=inf  Measurements=off
  IGBT/Diode1 : spsIGBTDiodeLib/IGBT//Diode  Ron=1e-3  Rs=1e5  Cs=inf  Measurements=off
  NOT : Logic  Operator=NOT  IconShape=distinctive  AllPortsSameDT=off  OutDataTypeStr=boolean
  Series RLC Branch : spsSeriesRLCBranchLib/Series RLC Branch  LConnTagsString=__new0  RConnTagsString=__new0  BranchType=C  Resistance=1  Inductance=1e-3  SetiL0=off  InitialCurrent=0  Capacitance=C_sm  Setx0=on  InitialVoltage=V_sm  Measurements=None
  Voltage Measurement : spsVoltageMeasurementLib/Voltage Measurement  PhasorSimulation=off  OutputType=Complex  PSBequivalent=0
  1 : PMIOPort  Side=Right
  2 : PMIOPort  Port=2  Side=Right
  tag scope: Vcup_sm1=global
  wires:
  NOT/1 -> IGBT/Diode1/1
  g/1 -> IGBT/Diode/1, NOT/1
  Voltage Measurement/1 -> [Vcup_sm1]
  connections:
  IGBT/Diode/RConn1 -- 1/RConn1 -- IGBT/Diode1/LConn1
  Series RLC Branch/LConn1 -- IGBT/Diode/LConn1 -- Voltage Measurement/LConn1
  Series RLC Branch/RConn1 -- 2/RConn1 -- IGBT/Diode1/RConn1 -- Voltage Measurement/LConn2

== system Assignment3_2_MMC/Subsystem13 ==
  g : Inport
  IGBT/Diode : spsIGBTDiodeLib/IGBT//Diode  Ron=1e-3  Rs=1e5  Cs=inf  Measurements=off
  IGBT/Diode1 : spsIGBTDiodeLib/IGBT//Diode  Ron=1e-3  Rs=1e5  Cs=inf  Measurements=off
  NOT : Logic  Operator=NOT  IconShape=distinctive  AllPortsSameDT=off  OutDataTypeStr=boolean
  Series RLC Branch : spsSeriesRLCBranchLib/Series RLC Branch  LConnTagsString=__new0  RConnTagsString=__new0  BranchType=C  Resistance=1  Inductance=1e-3  SetiL0=off  InitialCurrent=0  Capacitance=C_sm  Setx0=on  InitialVoltage=V_sm  Measurements=None
  Voltage Measurement : spsVoltageMeasurementLib/Voltage Measurement  PhasorSimulation=off  OutputType=Complex  PSBequivalent=0
  1 : PMIOPort  Side=Right
  2 : PMIOPort  Port=2  Side=Right
  tag scope: Vcup_sm2=global
  wires:
  NOT/1 -> IGBT/Diode1/1
  g/1 -> IGBT/Diode/1, NOT/1
  Voltage Measurement/1 -> [Vcup_sm2]
  connections:
  IGBT/Diode/RConn1 -- 1/RConn1 -- IGBT/Diode1/LConn1
  Series RLC Branch/LConn1 -- IGBT/Diode/LConn1 -- Voltage Measurement/LConn1
  Series RLC Branch/RConn1 -- 2/RConn1 -- IGBT/Diode1/RConn1 -- Voltage Measurement/LConn2

== system Assignment3_2_MMC/Subsystem14 ==
  g : Inport
  IGBT/Diode : spsIGBTDiodeLib/IGBT//Diode  Ron=1e-3  Rs=1e5  Cs=inf  Measurements=off
  IGBT/Diode1 : spsIGBTDiodeLib/IGBT//Diode  Ron=1e-3  Rs=1e5  Cs=inf  Measurements=off
  NOT : Logic  Operator=NOT  IconShape=distinctive  AllPortsSameDT=off  OutDataTypeStr=boolean
  Series RLC Branch : spsSeriesRLCBranchLib/Series RLC Branch  LConnTagsString=__new0  RConnTagsString=__new0  BranchType=C  Resistance=1  Inductance=1e-3  SetiL0=off  InitialCurrent=0  Capacitance=C_sm  Setx0=on  InitialVoltage=V_sm  Measurements=None
  Voltage Measurement : spsVoltageMeasurementLib/Voltage Measurement  PhasorSimulation=off  OutputType=Complex  PSBequivalent=0
  1 : PMIOPort  Side=Right
  2 : PMIOPort  Port=2  Side=Right
  tag scope: Vcup_sm3=global
  wires:
  NOT/1 -> IGBT/Diode1/1
  g/1 -> IGBT/Diode/1, NOT/1
  Voltage Measurement/1 -> [Vcup_sm3]
  connections:
  IGBT/Diode/RConn1 -- 1/RConn1 -- IGBT/Diode1/LConn1
  Series RLC Branch/LConn1 -- IGBT/Diode/LConn1 -- Voltage Measurement/LConn1
  Series RLC Branch/RConn1 -- 2/RConn1 -- IGBT/Diode1/RConn1 -- Voltage Measurement/LConn2

== system Assignment3_2_MMC/Subsystem15 ==
  g : Inport
  IGBT/Diode : spsIGBTDiodeLib/IGBT//Diode  Ron=1e-3  Rs=1e5  Cs=inf  Measurements=off
  IGBT/Diode1 : spsIGBTDiodeLib/IGBT//Diode  Ron=1e-3  Rs=1e5  Cs=inf  Measurements=off
  NOT : Logic  Operator=NOT  IconShape=distinctive  AllPortsSameDT=off  OutDataTypeStr=boolean
  Series RLC Branch : spsSeriesRLCBranchLib/Series RLC Branch  LConnTagsString=__new0  RConnTagsString=__new0  BranchType=C  Resistance=1  Inductance=1e-3  SetiL0=off  InitialCurrent=0  Capacitance=C_sm  Setx0=on  InitialVoltage=V_sm  Measurements=None
  Voltage Measurement : spsVoltageMeasurementLib/Voltage Measurement  PhasorSimulation=off  OutputType=Complex  PSBequivalent=0
  1 : PMIOPort  Side=Right
  2 : PMIOPort  Port=2  Side=Right
  tag scope: Vcup_sm4=global
  wires:
  NOT/1 -> IGBT/Diode1/1
  g/1 -> IGBT/Diode/1, NOT/1
  Voltage Measurement/1 -> [Vcup_sm4]
  connections:
  IGBT/Diode/RConn1 -- 1/RConn1 -- IGBT/Diode1/LConn1
  Series RLC Branch/LConn1 -- IGBT/Diode/LConn1 -- Voltage Measurement/LConn1
  Series RLC Branch/RConn1 -- 2/RConn1 -- IGBT/Diode1/RConn1 -- Voltage Measurement/LConn2

== system Assignment3_2_MMC/Subsystem16 ==
  g : Inport
  IGBT/Diode : spsIGBTDiodeLib/IGBT//Diode  Ron=1e-3  Rs=1e5  Cs=inf  Measurements=off
  IGBT/Diode1 : spsIGBTDiodeLib/IGBT//Diode  Ron=1e-3  Rs=1e5  Cs=inf  Measurements=off
  NOT : Logic  Operator=NOT  IconShape=distinctive  AllPortsSameDT=off  OutDataTypeStr=boolean
  Series RLC Branch : spsSeriesRLCBranchLib/Series RLC Branch  LConnTagsString=__new0  RConnTagsString=__new0  BranchType=C  Resistance=1  Inductance=1e-3  SetiL0=off  InitialCurrent=0  Capacitance=C_sm  Setx0=on  InitialVoltage=V_sm  Measurements=None
  Voltage Measurement : spsVoltageMeasurementLib/Voltage Measurement  PhasorSimulation=off  OutputType=Complex  PSBequivalent=0
  1 : PMIOPort  Side=Right
  2 : PMIOPort  Port=2  Side=Right
  tag scope: Vblow_sm1=global
  wires:
  NOT/1 -> IGBT/Diode1/1
  g/1 -> IGBT/Diode/1, NOT/1
  Voltage Measurement/1 -> [Vblow_sm1]
  connections:
  IGBT/Diode/RConn1 -- 1/RConn1 -- IGBT/Diode1/LConn1
  Series RLC Branch/LConn1 -- IGBT/Diode/LConn1 -- Voltage Measurement/LConn1
  Series RLC Branch/RConn1 -- 2/RConn1 -- IGBT/Diode1/RConn1 -- Voltage Measurement/LConn2

== system Assignment3_2_MMC/Subsystem17 ==
  g : Inport
  IGBT/Diode : spsIGBTDiodeLib/IGBT//Diode  Ron=1e-3  Rs=1e5  Cs=inf  Measurements=off
  IGBT/Diode1 : spsIGBTDiodeLib/IGBT//Diode  Ron=1e-3  Rs=1e5  Cs=inf  Measurements=off
  NOT : Logic  Operator=NOT  IconShape=distinctive  AllPortsSameDT=off  OutDataTypeStr=boolean
  Series RLC Branch : spsSeriesRLCBranchLib/Series RLC Branch  LConnTagsString=__new0  RConnTagsString=__new0  BranchType=C  Resistance=1  Inductance=1e-3  SetiL0=off  InitialCurrent=0  Capacitance=C_sm  Setx0=on  InitialVoltage=V_sm  Measurements=None
  Voltage Measurement : spsVoltageMeasurementLib/Voltage Measurement  PhasorSimulation=off  OutputType=Complex  PSBequivalent=0
  1 : PMIOPort  Side=Right
  2 : PMIOPort  Port=2  Side=Right
  tag scope: Vblow_sm2=global
  wires:
  NOT/1 -> IGBT/Diode1/1
  g/1 -> IGBT/Diode/1, NOT/1
  Voltage Measurement/1 -> [Vblow_sm2]
  connections:
  IGBT/Diode/RConn1 -- 1/RConn1 -- IGBT/Diode1/LConn1
  Series RLC Branch/LConn1 -- IGBT/Diode/LConn1 -- Voltage Measurement/LConn1
  Series RLC Branch/RConn1 -- 2/RConn1 -- IGBT/Diode1/RConn1 -- Voltage Measurement/LConn2

== system Assignment3_2_MMC/Subsystem18 ==
  g : Inport
  IGBT/Diode : spsIGBTDiodeLib/IGBT//Diode  Ron=1e-3  Rs=1e5  Cs=inf  Measurements=off
  IGBT/Diode1 : spsIGBTDiodeLib/IGBT//Diode  Ron=1e-3  Rs=1e5  Cs=inf  Measurements=off
  NOT : Logic  Operator=NOT  IconShape=distinctive  AllPortsSameDT=off  OutDataTypeStr=boolean
  Series RLC Branch : spsSeriesRLCBranchLib/Series RLC Branch  LConnTagsString=__new0  RConnTagsString=__new0  BranchType=C  Resistance=1  Inductance=1e-3  SetiL0=off  InitialCurrent=0  Capacitance=C_sm  Setx0=on  InitialVoltage=V_sm  Measurements=None
  Voltage Measurement : spsVoltageMeasurementLib/Voltage Measurement  PhasorSimulation=off  OutputType=Complex  PSBequivalent=0
  1 : PMIOPort  Side=Right
  2 : PMIOPort  Port=2  Side=Right
  tag scope: Vblow_sm3=global
  wires:
  NOT/1 -> IGBT/Diode1/1
  g/1 -> IGBT/Diode/1, NOT/1
  Voltage Measurement/1 -> [Vblow_sm3]
  connections:
  IGBT/Diode/RConn1 -- 1/RConn1 -- IGBT/Diode1/LConn1
  Series RLC Branch/LConn1 -- IGBT/Diode/LConn1 -- Voltage Measurement/LConn1
  Series RLC Branch/RConn1 -- 2/RConn1 -- IGBT/Diode1/RConn1 -- Voltage Measurement/LConn2

== system Assignment3_2_MMC/Subsystem19 ==
  g : Inport
  IGBT/Diode : spsIGBTDiodeLib/IGBT//Diode  Ron=1e-3  Rs=1e5  Cs=inf  Measurements=off
  IGBT/Diode1 : spsIGBTDiodeLib/IGBT//Diode  Ron=1e-3  Rs=1e5  Cs=inf  Measurements=off
  NOT : Logic  Operator=NOT  IconShape=distinctive  AllPortsSameDT=off  OutDataTypeStr=boolean
  Series RLC Branch : spsSeriesRLCBranchLib/Series RLC Branch  LConnTagsString=__new0  RConnTagsString=__new0  BranchType=C  Resistance=1  Inductance=1e-3  SetiL0=off  InitialCurrent=0  Capacitance=C_sm  Setx0=on  InitialVoltage=V_sm  Measurements=None
  Voltage Measurement : spsVoltageMeasurementLib/Voltage Measurement  PhasorSimulation=off  OutputType=Complex  PSBequivalent=0
  1 : PMIOPort  Side=Right
  2 : PMIOPort  Port=2  Side=Right
  tag scope: Vblow_sm4=global
  wires:
  NOT/1 -> IGBT/Diode1/1
  g/1 -> IGBT/Diode/1, NOT/1
  Voltage Measurement/1 -> [Vblow_sm4]
  connections:
  IGBT/Diode/RConn1 -- 1/RConn1 -- IGBT/Diode1/LConn1
  Series RLC Branch/LConn1 -- IGBT/Diode/LConn1 -- Voltage Measurement/LConn1
  Series RLC Branch/RConn1 -- 2/RConn1 -- IGBT/Diode1/RConn1 -- Voltage Measurement/LConn2

== system Assignment3_2_MMC/Subsystem2 ==
  g : Inport
  IGBT/Diode : spsIGBTDiodeLib/IGBT//Diode  Ron=1e-3  Rs=1e5  Cs=inf  Measurements=off
  IGBT/Diode1 : spsIGBTDiodeLib/IGBT//Diode  Ron=1e-3  Rs=1e5  Cs=inf  Measurements=off
  NOT : Logic  Operator=NOT  IconShape=distinctive  AllPortsSameDT=off  OutDataTypeStr=boolean
  Series RLC Branch : spsSeriesRLCBranchLib/Series RLC Branch  LConnTagsString=__new0  RConnTagsString=__new0  BranchType=C  Resistance=1  Inductance=1e-3  SetiL0=off  InitialCurrent=0  Capacitance=C_sm  Setx0=on  InitialVoltage=V_sm  Measurements=None
  Voltage Measurement : spsVoltageMeasurementLib/Voltage Measurement  PhasorSimulation=off  OutputType=Complex  PSBequivalent=0
  1 : PMIOPort  Side=Right
  2 : PMIOPort  Port=2  Side=Right
  tag scope: Vaup_sm3=global
  wires:
  NOT/1 -> IGBT/Diode1/1
  g/1 -> IGBT/Diode/1, NOT/1
  Voltage Measurement/1 -> [Vaup_sm3]
  connections:
  IGBT/Diode/RConn1 -- 1/RConn1 -- IGBT/Diode1/LConn1
  Series RLC Branch/LConn1 -- IGBT/Diode/LConn1 -- Voltage Measurement/LConn1
  Series RLC Branch/RConn1 -- 2/RConn1 -- IGBT/Diode1/RConn1 -- Voltage Measurement/LConn2

== system Assignment3_2_MMC/Subsystem20 ==
  g : Inport
  IGBT/Diode : spsIGBTDiodeLib/IGBT//Diode  Ron=1e-3  Rs=1e5  Cs=inf  Measurements=off
  IGBT/Diode1 : spsIGBTDiodeLib/IGBT//Diode  Ron=1e-3  Rs=1e5  Cs=inf  Measurements=off
  NOT : Logic  Operator=NOT  IconShape=distinctive  AllPortsSameDT=off  OutDataTypeStr=boolean
  Series RLC Branch : spsSeriesRLCBranchLib/Series RLC Branch  LConnTagsString=__new0  RConnTagsString=__new0  BranchType=C  Resistance=1  Inductance=1e-3  SetiL0=off  InitialCurrent=0  Capacitance=C_sm  Setx0=on  InitialVoltage=V_sm  Measurements=None
  Voltage Measurement : spsVoltageMeasurementLib/Voltage Measurement  PhasorSimulation=off  OutputType=Complex  PSBequivalent=0
  1 : PMIOPort  Side=Right
  2 : PMIOPort  Port=2  Side=Right
  tag scope: Vclow_sm1=global
  wires:
  NOT/1 -> IGBT/Diode1/1
  g/1 -> IGBT/Diode/1, NOT/1
  Voltage Measurement/1 -> [Vclow_sm1]
  connections:
  IGBT/Diode/RConn1 -- 1/RConn1 -- IGBT/Diode1/LConn1
  Series RLC Branch/LConn1 -- IGBT/Diode/LConn1 -- Voltage Measurement/LConn1
  Series RLC Branch/RConn1 -- 2/RConn1 -- IGBT/Diode1/RConn1 -- Voltage Measurement/LConn2

== system Assignment3_2_MMC/Subsystem21 ==
  g : Inport
  IGBT/Diode : spsIGBTDiodeLib/IGBT//Diode  Ron=1e-3  Rs=1e5  Cs=inf  Measurements=off
  IGBT/Diode1 : spsIGBTDiodeLib/IGBT//Diode  Ron=1e-3  Rs=1e5  Cs=inf  Measurements=off
  NOT : Logic  Operator=NOT  IconShape=distinctive  AllPortsSameDT=off  OutDataTypeStr=boolean
  Series RLC Branch : spsSeriesRLCBranchLib/Series RLC Branch  LConnTagsString=__new0  RConnTagsString=__new0  BranchType=C  Resistance=1  Inductance=1e-3  SetiL0=off  InitialCurrent=0  Capacitance=C_sm  Setx0=on  InitialVoltage=V_sm  Measurements=None
  Voltage Measurement : spsVoltageMeasurementLib/Voltage Measurement  PhasorSimulation=off  OutputType=Complex  PSBequivalent=0
  1 : PMIOPort  Side=Right
  2 : PMIOPort  Port=2  Side=Right
  tag scope: Vclow_sm2=global
  wires:
  NOT/1 -> IGBT/Diode1/1
  g/1 -> IGBT/Diode/1, NOT/1
  Voltage Measurement/1 -> [Vclow_sm2]
  connections:
  IGBT/Diode/RConn1 -- 1/RConn1 -- IGBT/Diode1/LConn1
  Series RLC Branch/LConn1 -- IGBT/Diode/LConn1 -- Voltage Measurement/LConn1
  Series RLC Branch/RConn1 -- 2/RConn1 -- IGBT/Diode1/RConn1 -- Voltage Measurement/LConn2
